simulink model "synchronousGeneratorPLECS"  (R2016b)
settings: Solver=FixedStepAuto  StartTime=0.0  StopTime=0.3  FixedStep=0.00005  RelTol=1e-3
undefined symbols (not defined in the file or in its folder): plecs
settings Model: Creator=mmi-vsa  LastModifiedBy=mmi-vsa

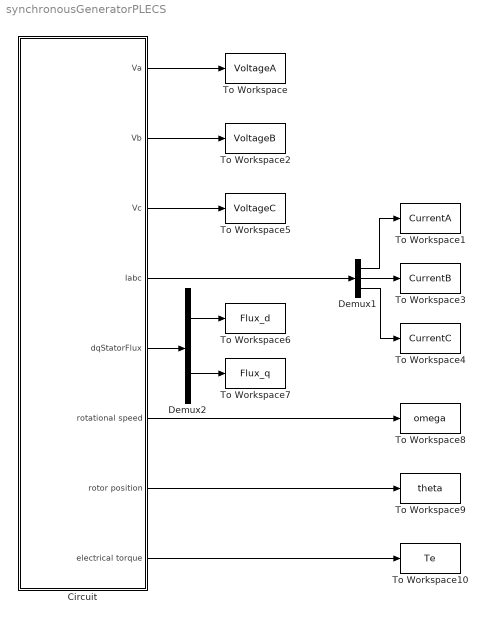
== system synchronousGeneratorPLECS ==
  Circuit : Subsystem  LoadFcn=plecs('sl', 200);  InitFcn=plecs('sl', 214);  StartFcn=plecs('sl', 208);  StopFcn=plecs('sl', 209);  mask(PlecsCircuit){PLECSData=<binary blob, 5384 chars, not shown>}
      mask prompts: PLECSData "PLECS Data (Do not delete or modify!)"
      mask init:
      | % PLACE CUSTOM INITIALIZATIONS ABOVE
      | % DO NOT REMOVE
      | plecs('sl', 215);
      | % DO NOT REMOVE
      settings: CopyFcn=plecs('sl', 203);  DeleteFcn=plecs('sl', 205);  UndoDeleteFcn=plecs('sl', 206);  PreSaveFcn=plecs('sl', 211);  PostSaveFcn=plecs('sl', 201);  NameChangeFcn=plecs('sl', 210);  DestroyFcn=plecs('sl', 207);  PreCopyFcn=plecs('sl', 216);  OpenFcn=plecs('sl', 202);  ErrorFcn=plerrorfcn
      mask Help: web(['file:///' fullfile(plecsdoc, 'creatingacircuit.html')])
      mask Display: disp('PLECS\nCircuit')
  Demux1 : Demux  Outputs=3
  Demux2 : Demux  Outputs=2
  To Workspace : ToWorkspace  VariableName=VoltageA  SampleTime=-1
  To Workspace1 : ToWorkspace  VariableName=CurrentA  SampleTime=-1
  To Workspace10 : ToWorkspace  VariableName=Te  SampleTime=-1
  To Workspace2 : ToWorkspace  VariableName=VoltageB  SampleTime=-1
  To Workspace3 : ToWorkspace  VariableName=CurrentB  SampleTime=-1
  To Workspace4 : ToWorkspace  VariableName=CurrentC  SampleTime=-1
  To Workspace5 : ToWorkspace  VariableName=VoltageC  SampleTime=-1
  To Workspace6 : ToWorkspace  VariableName=Flux_d  SampleTime=-1
  To Workspace7 : ToWorkspace  VariableName=Flux_q  SampleTime=-1
  To Workspace8 : ToWorkspace  VariableName=omega  SampleTime=-1
  To Workspace9 : ToWorkspace  VariableName=theta  SampleTime=-1
  wires:
  Demux1/1 -> To Workspace1/1
  Demux1/2 -> To Workspace3/1
  Demux1/3 -> To Workspace4/1
  Circuit/1(Va) -> To Workspace/1
  Circuit/2(Vb) -> To Workspace2/1
  Circuit/3(Vc) -> To Workspace5/1
  Circuit/4(Iabc) -> Demux1/1
  Circuit/5(dqStatorFlux) -> Demux2/1
  Demux2/1 -> To Workspace6/1
  Demux2/2 -> To Workspace7/1
  Circuit/6(rotational speed) -> To Workspace8/1
  Circuit/7(rotor position) -> To Workspace9/1
  Circuit/8(electrical torque) -> To Workspace10/1

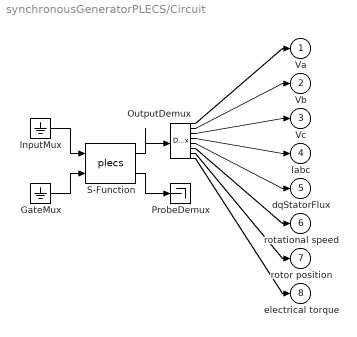
== system synchronousGeneratorPLECS/Circuit ==
  " GateMux " : Ground
  " InputMux " : Ground
  " OutputDemux " : Demux  Outputs=[ 1 1 1 3 2 1 1 1 ]
  " ProbeDemux " : Terminator
  " S-Function " : S-Function  FunctionName=plecs  SFunctionDeploymentMode=off  EnableBusSupport=off
  Va : Outport  PortDimensions=1
  Vb : Outport  Port=2  PortDimensions=1
  Vc : Outport  Port=3  PortDimensions=1
  Iabc : Outport  Port=4  PortDimensions=3
  dqStatorFlux : Outport  Port=5  PortDimensions=2
  rotational speed : Outport  Port=6  PortDimensions=1
  rotor position : Outport  Port=7  PortDimensions=1
  electrical torque : Outport  Port=8  PortDimensions=1
  wires:
  " S-Function "/1 -> " OutputDemux "/1
  " InputMux "/1 -> " S-Function "/1
  " GateMux "/1 -> " S-Function "/2
  " S-Function "/2 -> " ProbeDemux "/1
  " OutputDemux "/1 -> Va/1
  " OutputDemux "/2 -> Vb/1
  " OutputDemux "/3 -> Vc/1
  " OutputDemux "/4 -> Iabc/1
  " OutputDemux "/5 -> dqStatorFlux/1
  " OutputDemux "/6 -> rotational speed/1
  " OutputDemux "/7 -> rotor position/1
  " OutputDemux "/8 -> electrical torque/1
